simulink model "FMCW_chirp_generator_Rev00"  (R2021b)
settings: Solver=VariableStepAuto  StartTime=0.0  StopTime=30  RelTol=1e-3
values from neighbouring files (symbols this model uses):
  chirp = [zeros(chirp_params.num_samples_idle_time,1); waveform()]    [sensing_system_revA_performance_evaluation.m]
  chirps = obj.chirps    [Radar_revA.m]
undefined symbols (not defined in the file or in its folder): active_frame_time, frame_cycle_time
libraries: hdlsllib x2, simulink x1
settings Model: Creator=David  LastModifiedBy=David

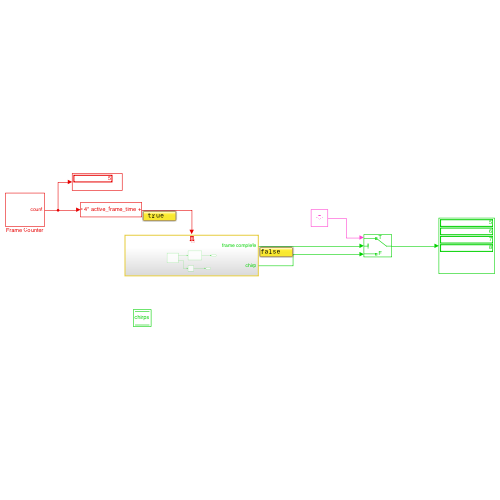
[thumbnail: Simulink's stored preview of the top-level diagram]
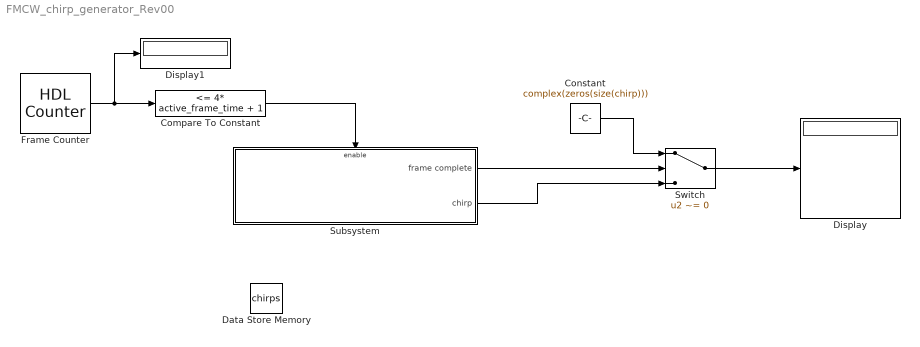
== system FMCW_chirp_generator_Rev00 ==
  Compare To Constant : simulink/Logic and Bit Operations/Compare To Constant  relop=<=  const=4* active_frame_time + 1  OutDataTypeStr=boolean
  Constant : Constant  Value=complex(zeros(size(chirp)))  VectorParams1D=off
  Data Store Memory : DataStoreMemory  DataStoreName=chirps  ReadBeforeWriteMsg=warning  WriteAfterWriteMsg=warning  WriteAfterReadMsg=warning  InitialValue=chirps  ShowAdditionalParam=off  OutDataTypeStr=double  Dimensions=size(chirps)
      settings: SignalType=complex
  Display : Display
  Display1 : Display
  Frame Counter : hdlsllib/Sources/HDL Counter  CountType=Count limited  CountInit=1  CountStep=1  CountMax=4*frame_cycle_time  CountFromType=Initial value  CountFrom=1  CountResetPort=off  CountLoadPort=off  CountEnbPort=off  CountDirPort=off  CountHitOutputPort=off  CountDataType=Unsigned  CountWordLen=8  CountFracLen=0  CountSampTime=0.25
  Subsystem : Subsystem
  Switch : Switch  Criteria=u2 ~= 0
  wires:
  Frame Counter/1 -> Compare To Constant/1, Display1/1
  Compare To Constant/1 -> Subsystem/Enable
  Constant/1 -> Switch/1
  Subsystem/2(chirp) -> Switch/3
  Switch/1 -> Display/1
  Subsystem/1(frame complete) -> Switch/2

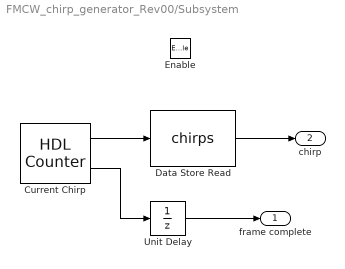
== system FMCW_chirp_generator_Rev00/Subsystem ==
  Enable : EnablePort  StatesWhenEnabling=reset
  Current Chirp : hdlsllib/Sources/HDL Counter  CountType=Count limited  CountInit=1  CountStep=1  CountMax=num_chirps  CountFromType=Initial value  CountFrom=1  CountResetPort=off  CountLoadPort=off  CountEnbPort=off  CountDirPort=off  CountHitOutputPort=on  CountDataType=Unsigned  CountWordLen=8  CountFracLen=0  CountSampTime=chirp_cycle_time
  Data Store Read : DataStoreRead  DataStoreName=chirps  DataStoreElements=chirps  EnableIndexing=on  NumberOfDimensions=2  IndexOptions=Index vector (port),Select all  Indices=1,1  OutputSizes=1,1
  Unit Delay : UnitDelay  SampleTime=-1  HasFrameUpgradeWarning=on
  frame complete : Outport
  chirp : Outport  Port=2
  wires:
  Current Chirp/1 -> Data Store Read/1
  Current Chirp/2 -> Unit Delay/1
  Data Store Read/1 -> chirp/1
  Unit Delay/1 -> frame complete/1
